simulink model "PV_ANN1"  (R2024b)
settings: Solver=ode23tb  StartTime=0.0  StopTime=3  MaxStep=1e-4  RelTol=1e-3
values from neighbouring files (symbols this model uses):
  TestID = testIDs(k)    [CloudMPPT_FullAnalytics.m]    (also in TestID.m = 0)
undefined symbols (not defined in the file or in its folder): MCS_ML_Selector_fun, sigbuilder_block
libraries: spsSeriesRLCBranchLib x3, spsDiodeLib x2, spsVoltageMeasurementLib x2, spsCurrentMeasurementLib x1, spsControlledCurrentSourceLib x1, spsIGBTLib x1, sps_lib x1, spsPWMGeneratorDCDCLib x1
(part 1 of 2)
settings Model: SimulationMode=accelerator  Creator=Ankita Arora  LastModifiedBy=qazvin
settings SolverCC: ZeroCrossAlgorithm=Adaptive  AlgebraicLoopSolver=TrustRegion
settings DataIOCC: SaveState=on  SignalLogging=off  ReturnWorkspaceOutputs=off
settings OptimizationCC: LifeSpan=inf
settings DebuggingCC: UnconnectedInputMsg=warning  UnconnectedOutputMsg=warning  UnconnectedLineMsg=warning  SFExecutionAtInitializationDiag=none  ArithmeticOperatorsInVariantConditions=warning
settings ModelReferenceCC: EnableRefExpFcnMdlSchedulingChecks=on
settings SFSimCC: SimUseLocalCustomCode=off  CustomCodeUndefinedFunction=UseInterfaceOnly
settings RTWCC: RTWUseLocalCustomCode=off  GPUComputeCapability=3.5
settings CodeAppCC: StateflowObjectComments=on
settings SimscapeCC: SimscapeNormalizeSystem=off

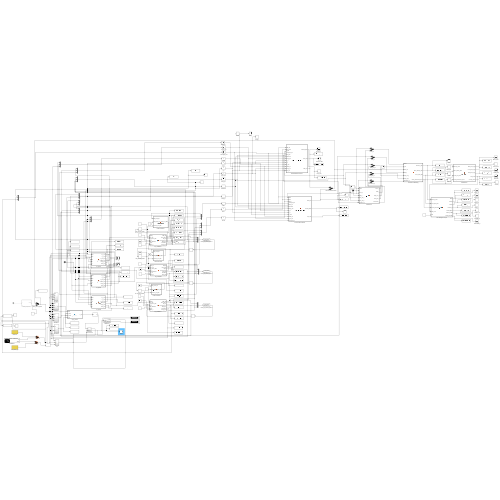
[thumbnail: Simulink's stored preview of the top-level diagram]
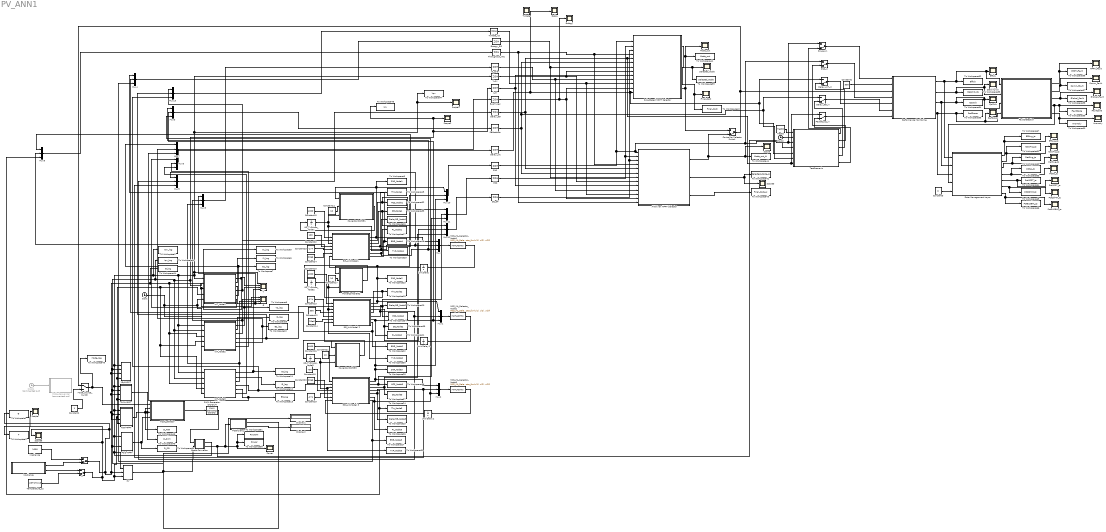
== system PV_ANN1 ==
  "      " : ManualSwitch  CurrentSetting=0
  "      1" : ManualSwitch  CurrentSetting=0
  " PacketLoss_in" : ManualSwitch  CurrentSetting=0
  " StabilityIdx   " : Scope
  5G_LinkModel 2 : MATLAB Function  TreatAsAtomicUnit=on
  "5G_LinkModel 3 " : MATLAB Function  TreatAsAtomicUnit=on
  "5G_LinkModel1 " : MATLAB Function  TreatAsAtomicUnit=on
  AI-Driven MPPT Selector : MATLAB Function  TreatAsAtomicUnit=on  SystemSampleTime=1e-4
  ANN-MPPT : Subsystem
  Anomaly : Scope
  Boost Convertor : Subsystem
  Clock : Clock
  Clock1 : Clock  Commented=on
  Clock2 : Clock
  Comm_Fault : Scope
  Constant1 : Constant
  Constant10 : Constant  Value=4000
  Constant11 : Constant  Value=10
  Constant12 : Constant  Value=300
  Constant13 : Constant  Value=-174
  Constant14 : Constant  Value=20e6
  Constant15 : Constant  Value=4000
  Constant16 : Constant  Value=4000
  Constant17 : Constant  Value=10
  Constant18 : Constant  Value=700
  Constant19 : Constant  Value=-174
  Constant2 : Constant  Value=500
  Constant20 : Constant  Value=20e6
  Constant21 : Constant  Value=10
  Constant22 : Constant  Value=100
  Constant23 : Constant  Value=-174
  Constant24 : Constant  Value=20e6
  Constant3 : Constant  Value=0
  Controller Selector Switch : ManualSwitch  CurrentSetting=0
  Data Management Layer : MATLAB Function  TreatAsAtomicUnit=on
  Delay : Scope
  Delay_5G : ZeroOrderHold  SampleTime=0.1
  Delay_5G_in : ManualSwitch  CurrentSetting=0
  Delay_IoT_in : ManualSwitch  CurrentSetting=0
  Delay_iot : ZeroOrderHold  SampleTime=0.1
  Display1 : Display
  Display2 : Display
  E_IoT_Vec : ZeroOrderHold  SampleTime=0.1
  EffAvg_ts : Scope
  EffIdx : Scope
  Energy : Scope
  Energy_5G : ZeroOrderHold  SampleTime=0.1
  FaultCode : Scope
  FaultDetection : MATLAB Function  TreatAsAtomicUnit=on
  Final_Cost : Scope
  G : Scope  NumInputPorts=4
  G_solar : ZeroOrderHold  SampleTime=0.1
  Global_Fault : Scope
  I_pv : ZeroOrderHold  SampleTime=0.1
  IoT_Node1 : MATLAB Function  TreatAsAtomicUnit=on  SystemSampleTime=0.01
  IoT_Node2 : MATLAB Function  TreatAsAtomicUnit=on  SystemSampleTime=0.02
  IoT_Node3 : MATLAB Function  TreatAsAtomicUnit=on  SystemSampleTime=0.05
  Irradiance : Constant  Value=1000
  "Irradiance " : Subsystem  Tag=STV Subsys  LoadFcn=sigbuilder_block('load');  StartFcn=sigbuilder_block('start');  StopFcn=sigbuilder_block('stop');  ClipboardFcn=sigbuilder_block('clipboard');  mask(Sigbuilder block){tuvar=[0:10]}
      mask help: Sigbuilder GUI
      mask init:
      | if ~strcmp(get_param(bdroot(gcbh),'SimulationStatus'),'stopped') tuvar = sigbuilder_block('maskInit'); end
      settings: CopyFcn=sigbuilder_block('copy');  DeleteFcn=sigbuilder_block('delete');  ModelCloseFcn=sigbuilder_block('modelClose');  PreSaveFcn=sigbuilder_block('preSave');  PauseFcn=sigbuilder_block('pause')  ContinueFcn=sigbuilder_block('continue')  NameChangeFcn=sigbuilder_block('namechange');  OpenFcn=sigbuilder_block('open',[5.4 30 1141.2 507.6 ]);  CloseFcn=sigbuilder_block('close');
      mask Display: plot(0, 0, 100, 100,[2, 2, 32, 32, 2], [68, 8, 8, 68, 68],[32, 2], [38, 38], [32, 19, 2],[53, 60, 44], [32, 17, 17, 2],[16, 16, 31, 31]);txt = getActiveGroup(gcbh);text(2, 100, txt,'verticalAlignment', 'top');
  MCS : ZeroOrderHold  SampleTime=0.1
  MCS_ML_Selector_Node1 : MATLABFcn  MATLABFcn=MCS_ML_Selector_fun(u(1), u(2), u(3))
  MCS_ML_Selector_Node2 : MATLABFcn  MATLABFcn=MCS_ML_Selector_fun(u(1), u(2), u(3))
  MCS_ML_Selector_Node3 : MATLABFcn  MATLABFcn=MCS_ML_Selector_fun(u(1), u(2), u(3))
  MPPT_Fault : Scope
  Mode_Sequencer : MATLAB Function  Commented=on  TreatAsAtomicUnit=on
  Mode_Source_Switch : ManualSwitch
  Mode_out : Scope
  Mux{,1..13} (14 alike) : Mux  Inputs=3
  P&Eficiency : Subsystem
  P&O-MPPT : Subsystem
  PV : Subsystem
  PWM Generator (DC-DC)4 : spsPWMGeneratorDCDCLib/PWM Generator (DC-DC)  Fsw=5000  Ts=0
  PacketLost : ZeroOrderHold  SampleTime=0.1
  PctCOMM_ts : Scope
  PctGLOBAL_ts : Scope
  PctMPPT_ts : Scope
  PctNo_ts : Scope
  PerfAvg_ts : Scope
  PerfScore : Scope
  Performance Monitoring : MATLAB Function  TreatAsAtomicUnit=on  SystemSampleTime=1e-4
  Power : Scope
  PowerControl5G1 : MATLAB Function  TreatAsAtomicUnit=on
  PowerControl5G2 : MATLAB Function  TreatAsAtomicUnit=on
  PowerControl5G3 : MATLAB Function  TreatAsAtomicUnit=on
  Power_in : ManualSwitch  CurrentSetting=0
  QoSAvg_ts : Scope
  QoSIdx : Scope
  Rule-Based MPPT Selector : MATLAB Function  TreatAsAtomicUnit=on  SystemSampleTime=1e-4
  SE_eff : ZeroOrderHold  SampleTime=0.1
  SNR : ZeroOrderHold  SampleTime=0.1
  SNR_in : ManualSwitch  CurrentSetting=0
  SVM-MPPT : Subsystem
  Scope{,1..3,6..7} (6 alike) : Scope
  Selected_Node : Scope
  Temperature_op : Constant  Value=25+273.15
  TestID : Constant  Value=TestID
  TestScenario : MATLAB Function  TreatAsAtomicUnit=on  SystemSampleTime=1e-4
  Throughput_Vec : ZeroOrderHold  SampleTime=0.1
  To Workspace : ToWorkspace  VariableName=G  SaveFormat=Timeseries  SampleTime=-1
  To Workspace1 : ToWorkspace  VariableName=T  SaveFormat=Timeseries  SampleTime=-1
  To Workspace10 : ToWorkspace  VariableName=E2_log  SampleTime=-1
  To Workspace11 : ToWorkspace  VariableName=V3_log  SampleTime=-1
  To Workspace12 : ToWorkspace  VariableName=I3_log  SampleTime=-1
  To Workspace13 : ToWorkspace  VariableName=E3_log  SampleTime=-1
  To Workspace14 : ToWorkspace  VariableName=G_log  SampleTime=-1
  To Workspace15 : ToWorkspace  VariableName=Thr_Node1  SampleTime=-1
  To Workspace16 : ToWorkspace  VariableName=Delay5G_Node1  SampleTime=-1
  To Workspace17 : ToWorkspace  VariableName=PL_Node1  SampleTime=-1
  To Workspace18 : ToWorkspace  VariableName=E5G_Node1  SampleTime=-1
  To Workspace19 : ToWorkspace  VariableName=Thr_Node2  SampleTime=-1
  To Workspace2 : ToWorkspace  VariableName=Vpv_log  SampleTime=-1
  To Workspace20 : ToWorkspace  VariableName=Delay5G_Node2  SampleTime=-1
  To Workspace21 : ToWorkspace  VariableName=PL_Node2  SampleTime=-1
  To Workspace22 : ToWorkspace  VariableName=E5G_Node2  SampleTime=-1
  To Workspace23 : ToWorkspace  VariableName=SNR_Node2  SampleTime=-1
  To Workspace24 : ToWorkspace  VariableName=Thr_Node3  SampleTime=-1
  To Workspace25 : ToWorkspace  VariableName=Delay5G_Node3  SampleTime=-1
  To Workspace26 : ToWorkspace  VariableName=PL_Node3  SampleTime=-1
  To Workspace27 : ToWorkspace  VariableName=E5G_Node3  SampleTime=-1
  To Workspace28 : ToWorkspace  VariableName=SNR_Node3  SampleTime=-1
  To Workspace29 : ToWorkspace  VariableName=TxP_Node1  SampleTime=-1
  To Workspace3 : ToWorkspace  VariableName=SNR_Node1  SampleTime=-1
  To Workspace30 : ToWorkspace  VariableName=TxP_Node2  SampleTime=-1
  To Workspace31 : ToWorkspace  VariableName=TxP_Node3  SampleTime=-1
  To Workspace32 : ToWorkspace  VariableName=MCS_Node1  SampleTime=-1
  To Workspace33 : ToWorkspace  VariableName=SE_Node1  SampleTime=-1
  To Workspace34 : ToWorkspace  VariableName=MCS_Node2  SampleTime=-1
  To Workspace35 : ToWorkspace  VariableName=SE_Node2  SampleTime=-1
  To Workspace36 : ToWorkspace  VariableName=MCS_Node3  SampleTime=-1
  To Workspace37 : ToWorkspace  VariableName=SE_Node3  SampleTime=-1
  To Workspace38 : ToWorkspace  VariableName=Power  SampleTime=5e-5
  To Workspace39 : ToWorkspace  VariableName=Selected_Node  SampleTime=-1
  To Workspace4 : ToWorkspace  VariableName=Ipv_log  SampleTime=-1
  To Workspace40 : ToWorkspace  VariableName=Final_Cost  SampleTime=-1
  To Workspace41 : ToWorkspace  VariableName=Mode_out  SampleTime=-1
  To Workspace42 : ToWorkspace  VariableName=Selected_Node_AI  SampleTime=-1
  To Workspace43 : ToWorkspace  VariableName=Final_Cost_AI  SampleTime=-1
  To Workspace44 : ToWorkspace  VariableName=Mode_out_AI  SampleTime=-1
  To Workspace45 : ToWorkspace  VariableName=Mode_log  SampleTime=-1
  To Workspace46 : ToWorkspace  VariableName=D_ANN  SampleTime=-1
  To Workspace47 : ToWorkspace  VariableName=Vpv  SaveFormat=Structure With Time  SampleTime=-1
  To Workspace48 : ToWorkspace  VariableName=Ipv  SaveFormat=Structure With Time  SampleTime=-1
  To Workspace49 : ToWorkspace  VariableName=D_SVM  SampleTime=-1
  To Workspace5 : ToWorkspace  VariableName=V1_log  SampleTime=-1
  To Workspace50 : ToWorkspace  VariableName=D_PO  SampleTime=-1
  To Workspace51 : ToWorkspace  VariableName=PowerAI  SampleTime=5e-5
  To Workspace52 : ToWorkspace  VariableName=EffIdx  SaveFormat=Timeseries  SampleTime=-1
  To Workspace53 : ToWorkspace  VariableName=StabilityIdx  SaveFormat=Timeseries  SampleTime=-1
  To Workspace54 : ToWorkspace  VariableName=QoSIdx  SaveFormat=Timeseries  SampleTime=-1
  To Workspace55 : ToWorkspace  VariableName=PerfScore  SaveFormat=Timeseries  SampleTime=-1
  To Workspace56 : ToWorkspace  VariableName=MPPT_Fault  SaveFormat=Timeseries  SampleTime=-1
  To Workspace57 : ToWorkspace  VariableName=Comm_Fault  SaveFormat=Timeseries  SampleTime=-1
  To Workspace58 : ToWorkspace  VariableName=Global_Fault  SaveFormat=Timeseries  SampleTime=-1
  To Workspace59 : ToWorkspace  VariableName=FaultCode  SaveFormat=Timeseries  SampleTime=-1
  To Workspace6 : ToWorkspace  VariableName=I1_log  SampleTime=-1
  To Workspace60 : ToWorkspace  VariableName=Anomaly  SaveFormat=Timeseries  SampleTime=-1
  To Workspace61 : ToWorkspace  VariableName=QoSAvg_ts  SaveFormat=Timeseries  SampleTime=-1
  To Workspace62 : ToWorkspace  VariableName=PerfAvg_ts  SaveFormat=Timeseries  SampleTime=-1
  To Workspace63 : ToWorkspace  VariableName=PctNo_ts  SaveFormat=Timeseries  SampleTime=-1
  To Workspace64 : ToWorkspace  VariableName=PctMPPT_ts  SaveFormat=Timeseries  SampleTime=-1
  To Workspace65 : ToWorkspace  VariableName=PctCOMM_ts  SaveFormat=Timeseries  SampleTime=-1
  To Workspace66 : ToWorkspace  VariableName=PctGLOBAL_ts  SaveFormat=Timeseries  SampleTime=-1
  To Workspace67 : ToWorkspace  VariableName=EffAvg_ts  SaveFormat=Timeseries  SampleTime=-1
  To Workspace7 : ToWorkspace  VariableName=E1_log  SampleTime=-1
  To Workspace8 : ToWorkspace  VariableName=V2_log  SampleTime=-1
  To Workspace9 : ToWorkspace  VariableName=I2_log  SampleTime=-1
  TxRate : Scope
  TxRate_iot : ZeroOrderHold  SampleTime=0.1
  UD_TxPower_Node1 : UnitDelay  SampleTime=-1  HasFrameUpgradeWarning=on
  UD_TxPower_Node2 : UnitDelay  SampleTime=-1  HasFrameUpgradeWarning=on
  UD_TxPower_Node3 : UnitDelay  SampleTime=-1  HasFrameUpgradeWarning=on
  Unit Delay : UnitDelay  SampleTime=-1  HasFrameUpgradeWarning=on
  Unit Delay1 : UnitDelay  SampleTime=-1  HasFrameUpgradeWarning=on
  Unit Delay2 : UnitDelay  SampleTime=-1  HasFrameUpgradeWarning=on
  V : Scope  NumInputPorts=4
  V5p-MPPT : Subsystem
  V_pv : ZeroOrderHold  SampleTime=0.1
  mppt_selector : MATLAB Function  TreatAsAtomicUnit=on
  wires:
  Temperature_op/1 -> "      1"/2
  Irradiance/1 -> "      "/1
  "      "/1 -> Scope6/1, To Workspace/1, PV/2(G), IoT_Node3/3(G), IoT_Node2/3(G), G/1, IoT_Node1/3(G), To Workspace14/1, V5p-MPPT/3(G), SVM-MPPT/3(G), ANN-MPPT/3(G)  "G"
  "      1"/1 -> To Workspace1/1, Scope7/1, PV/3(T), ANN-MPPT/4(T), IoT_Node3/4(T), IoT_Node2/4(T), IoT_Node1/4(T), V5p-MPPT/4(T), SVM-MPPT/4(T)  "T"
  PV/1(I) -> IoT_Node3/2(Ipv), IoT_Node2/2(Ipv), IoT_Node1/2(Ipv), To Workspace48/1, Scope2/1, I_pv/1, To Workspace4/1, V5p-MPPT/2(Ipv), SVM-MPPT/2(Ipv), ANN-MPPT/2(Ipv), P&O-MPPT/2(Ipv), Boost Convertor/2(s)
  P&O-MPPT/1(D) -> To Workspace50/1, mppt_selector/4(D_PO)
  mppt_selector/1(D_ref) -> PWM Generator (DC-DC)4/1
  Boost Convertor/1(v) -> PV/1(V), IoT_Node3/1(Vpv), IoT_Node2/1(Vpv), V/1, To Workspace47/1, Scope1/1, V_pv/1, IoT_Node1/1(Vpv), To Workspace2/1, V5p-MPPT/1(Vpv), SVM-MPPT/1(Vpv), ANN-MPPT/1(Vpv), P&O-MPPT/1(Vpv)
  PWM Generator (DC-DC)4/1 -> Boost Convertor/1(g)
  P&Eficiency/1(Pmax) -> Display1/1
  P&Eficiency/2(max_efficiency) -> Display2/1
  IoT_Node1/1(V_pv_iot1) -> V/2, To Workspace5/1
  IoT_Node2/1(V_pv_iot2) -> To Workspace8/1, V/3
  IoT_Node3/1(V_pv_iot3) -> To Workspace11/1, V/4
  IoT_Node1/3(G_solar_iot1) -> Mux9/1, G/4
  IoT_Node3/3(G_solar_iot3) -> Mux9/3, G/3
  IoT_Node2/3(G_solar_iot2) -> Mux9/2, G/2
  IoT_Node3/2(I_pv_iot3) -> To Workspace12/1
  IoT_Node3/5(Energy_iot3) -> To Workspace13/1, Mux7/3
  IoT_Node2/5(Energy_iot2) -> Mux7/2, To Workspace10/1
  IoT_Node2/2(I_pv_iot2) -> To Workspace9/1
  IoT_Node1/5(Energy_iot1) -> Mux7/1, To Workspace7/1
  IoT_Node1/2(I_pv_iot1) -> To Workspace6/1
  Clock/1 -> IoT_Node1/5(t), IoT_Node2/5(t), IoT_Node3/5(t)
  IoT_Node1/4(TxRate_iot1) -> Mux13/1, "5G_LinkModel1 "/2(IoT_rate)
  Constant18/1 -> "5G_LinkModel 3 "/4(d_m)
  Constant19/1 -> "5G_LinkModel 3 "/5(N0_dBmPerHz)
  Constant20/1 -> "5G_LinkModel 3 "/6(B_Hz)
  Constant15/1 -> "5G_LinkModel1 "/1(Data_in)
  Constant22/1 -> "5G_LinkModel1 "/4(d_m)
  Constant23/1 -> "5G_LinkModel1 "/5(N0_dBmPerHz)
  Constant24/1 -> "5G_LinkModel1 "/6(B_Hz)
  IoT_Node2/4(TxRate_iot2) -> Mux13/2, 5G_LinkModel 2/2(IoT_rate)
  Constant10/1 -> 5G_LinkModel 2/1(Data_in)
  Constant12/1 -> 5G_LinkModel 2/4(d_m)
  Constant13/1 -> 5G_LinkModel 2/5(N0_dBmPerHz)
  Constant14/1 -> 5G_LinkModel 2/6(B_Hz)
  IoT_Node3/4(TxRate_iot3) -> Mux13/3, "5G_LinkModel 3 "/2(IoT_rate)
  Constant16/1 -> "5G_LinkModel 3 "/1(Data_in)
  "5G_LinkModel1 "/1(SNR_dB) -> Mux/1, PowerControl5G1/1(SNR_meas_dB), To Workspace3/1, Mux10/1
  "5G_LinkModel1 "/5(Delay_5G) -> Mux5/1, Mux/2, To Workspace16/1
  "5G_LinkModel1 "/6(PacketLost) -> Mux/3, Mux3/1, To Workspace17/1
  "5G_LinkModel1 "/7(Energy_5G) -> Mux4/1, To Workspace18/1
  5G_LinkModel 2/1(SNR_dB) -> PowerControl5G2/1(SNR_meas_dB), Mux10/2, To Workspace23/1, Mux1/1
  5G_LinkModel 2/5(Delay_5G) -> Mux5/2, Mux1/2, To Workspace20/1
  5G_LinkModel 2/6(PacketLost) -> Mux3/2, Mux1/3, To Workspace21/1
  5G_LinkModel 2/7(Energy_5G) -> Mux4/2, To Workspace22/1
  "5G_LinkModel 3 "/7(Energy_5G) -> Mux4/3, To Workspace27/1
  "5G_LinkModel 3 "/6(PacketLost) -> Mux3/3, Mux2/3, To Workspace26/1
  "5G_LinkModel 3 "/5(Delay_5G) -> To Workspace25/1, Mux5/3, Mux2/2
  "5G_LinkModel 3 "/1(SNR_dB) -> Mux10/3, PowerControl5G3/1(SNR_meas_dB), To Workspace28/1, Mux2/1
  UD_TxPower_Node3/1 -> To Workspace31/1, "5G_LinkModel 3 "/3(Tx_Power_dBm), PowerControl5G3/3(TxPower_prev_dBm)
  UD_TxPower_Node1/1 -> To Workspace29/1, "5G_LinkModel1 "/3(Tx_Power_dBm), PowerControl5G1/3(TxPower_prev_dBm)
  UD_TxPower_Node2/1 -> To Workspace30/1, 5G_LinkModel 2/3(Tx_Power_dBm), PowerControl5G2/3(TxPower_prev_dBm)
  PowerControl5G3/1(TxPower_out_dBm) -> UD_TxPower_Node3/1
  PowerControl5G1/1(TxPower_out_dBm) -> UD_TxPower_Node1/1
  PowerControl5G2/1(TxPower_out_dBm) -> UD_TxPower_Node2/1
  Constant11/1 -> PowerControl5G1/2(SNR_target_dB)
  Constant17/1 -> PowerControl5G2/2(SNR_target_dB)
  Constant21/1 -> PowerControl5G3/2(SNR_target_dB)
  "5G_LinkModel1 "/4(Throughput_bps) -> Mux8/1, To Workspace15/1
  5G_LinkModel 2/4(Throughput_bps) -> Mux8/2, To Workspace19/1
  "5G_LinkModel 3 "/4(Throughput_bps) -> Mux8/3, To Workspace24/1
  "5G_LinkModel 3 "/2(MCS_index) -> Mux11/3, To Workspace36/1
  "5G_LinkModel 3 "/3(SE_eff) -> To Workspace37/1, Mux12/3
  5G_LinkModel 2/2(MCS_index) -> To Workspace34/1, Mux11/2
  "5G_LinkModel1 "/3(SE_eff) -> Mux12/1, To Workspace33/1
  "5G_LinkModel1 "/2(MCS_index) -> Mux11/1, To Workspace32/1
  Mux/1 -> MCS_ML_Selector_Node1/1
  Mux1/1 -> MCS_ML_Selector_Node2/1
  Mux2/1 -> MCS_ML_Selector_Node3/1
  MCS_ML_Selector_Node3/1 -> Unit Delay2/1
  MCS_ML_Selector_Node2/1 -> Unit Delay1/1
  MCS_ML_Selector_Node1/1 -> Unit Delay/1
  Unit Delay/1 -> "5G_LinkModel1 "/7(MCS_in)
  Unit Delay1/1 -> 5G_LinkModel 2/7(MCS_in)
  Unit Delay2/1 -> "5G_LinkModel 3 "/7(MCS_in)
  IoT_Node1/6(Delay_iot1) -> Mux6/1
  IoT_Node2/6(Delay_iot2) -> Mux6/2
  IoT_Node3/6(Delay_iot3) -> Mux6/3
  Mux7/1 -> E_IoT_Vec/1
  Mux4/1 -> Energy_5G/1
  Mux5/1 -> Delay_5G/1
  Mux3/1 -> PacketLost/1
  Mux8/1 -> Throughput_Vec/1
  ANN-MPPT/1(D) -> To Workspace46/1, mppt_selector/2(D_ANN)
  SVM-MPPT/1(D) -> To Workspace49/1, mppt_selector/3(D_SVM)
  I_pv/1 -> AI-Driven MPPT Selector/9(I_pv), Rule-Based MPPT Selector/9(I_pv)
  Throughput_Vec/1 -> AI-Driven MPPT Selector/13(Throughput_iot), AI-Driven MPPT Selector/4(Throughput_Vec), Rule-Based MPPT Selector/4(Throughput_bps)
  E_IoT_Vec/1 -> AI-Driven MPPT Selector/12(E_IoT_Vec), Rule-Based MPPT Selector/12(Energy_iot), Energy/1
  Energy_5G/1 -> AI-Driven MPPT Selector/7(Energy_5G), Rule-Based MPPT Selector/7(Energy_5G)
  V_pv/1 -> AI-Driven MPPT Selector/8(V_pv), Rule-Based MPPT Selector/8(V_pv)
  Mux9/1 -> G_solar/1
  G_solar/1 -> AI-Driven MPPT Selector/10(G_solar), Rule-Based MPPT Selector/10(G_solar)
  Delay_5G/1 -> AI-Driven MPPT Selector/5(Delay_5G), " PacketLoss_in"/1, TestScenario/7(PacketLoss_in), Rule-Based MPPT Selector/5(Delay_5G)
  Mux6/1 -> Delay_iot/1
  Delay_iot/1 -> Delay/1, TestScenario/5(Delay_IoT_in), Delay_IoT_in/1, Rule-Based MPPT Selector/13(Delay_iot)
  Mux10/1 -> SNR/1
  SNR/1 -> Rule-Based MPPT Selector/1(SNR_dB), SNR_in/1, TestScenario/4(SNR_in), AI-Driven MPPT Selector/1(SNR)
  Mux11/1 -> MCS/1
  MCS/1 -> Rule-Based MPPT Selector/2(MCS_index), AI-Driven MPPT Selector/2(MCS)
  5G_LinkModel 2/3(SE_eff) -> Mux12/2, To Workspace35/1
  Mux12/1 -> SE_eff/1
  SE_eff/1 -> Rule-Based MPPT Selector/3(SE_eff), AI-Driven MPPT Selector/3(SE_eff)
  Rule-Based MPPT Selector/3(Mode_out) -> Mode_out/1, To Workspace41/1, Controller Selector Switch/1
  Rule-Based MPPT Selector/2(Final_Cost) -> To Workspace40/1, Final_Cost/1
  "Irradiance "/1(G) -> "      "/2
  "Irradiance "/2(Temp) -> "      1"/1
  Mux13/1 -> TxRate_iot/1
  Rule-Based MPPT Selector/1(Selected_Node) -> To Workspace39/1, Selected_Node/1
  TxRate_iot/1 -> AI-Driven MPPT Selector/11(TxRate_iot), Rule-Based MPPT Selector/11(TxRate_iot)
  AI-Driven MPPT Selector/1(Mode_out) -> Controller Selector Switch/2, Scope/1, To Workspace44/1
  AI-Driven MPPT Selector/3(Final_Cost) -> To Workspace43/1
  AI-Driven MPPT Selector/2(Selected_Node) -> To Workspace42/1, Scope3/1
  Clock1/1 -> Mode_Sequencer/1(t)
  Controller Selector Switch/1 -> Performance Monitoring/3(Mode_out), Mode_Source_Switch/1
  Mode_Source_Switch/1 -> To Workspace45/1, mppt_selector/1(Mode)
  Constant1/1 -> Mode_Source_Switch/2
  Constant2/1 -> Performance Monitoring/2(P_ref)
  Performance Monitoring/1(Efficiency_Index) -> Data Management Layer/1(Efficiency_Index), FaultDetection/1(Efficiency_Index), EffIdx/1, To Workspace52/1
  Performance Monitoring/2(MPPT_Stability_Index) -> " StabilityIdx   "/1, FaultDetection/2(MPPT_Stability_Index), To Workspace53/1
  Performance Monitoring/3(Comm_QoS_Index) -> Data Management Layer/2(Comm_QoS_Index), FaultDetection/3(Comm_QoS_Index), QoSIdx/1, To Workspace54/1
  Performance Monitoring/4(Overall_Performance_Score) -> Data Management Layer/3(Overall_Performance_Score), PerfScore/1, FaultDetection/4(Overall_Performance_Score), To Workspace55/1
  FaultDetection/1(MPPT_Fault_Flag) -> To Workspace56/1, MPPT_Fault/1
  FaultDetection/2(Comm_Fault_Flag) -> Comm_Fault/1, To Workspace57/1
  FaultDetection/3(Global_Fault_Flag) -> Global_Fault/1, To Workspace58/1
  FaultDetection/4(Fault_Code) -> Data Management Layer/4(Fault_Code), FaultCode/1, To Workspace59/1
  FaultDetection/5(Anomaly_Score) -> Anomaly/1, To Workspace60/1
  PacketLost/1 -> Rule-Based MPPT Selector/6(PacketLost), TestScenario/6(Delay_5G_in), Delay_5G_in/1, AI-Driven MPPT Selector/6(PacketLost)
  TestID/1 -> TestScenario/1(TestID)
  Clock2/1 -> TestScenario/2(t)
  Power_in/1 -> Performance Monitoring/1(Power)
  Boost Convertor/2(PVPower) -> Power_in/1, TestScenario/3(Power_in), To Workspace51/1, To Workspace38/1, Power/1, P&Eficiency/1(P_out)
  TestScenario/1(Power_t) -> Power_in/2
  SNR_in/1 -> Performance Monitoring/4(SNR_in)
  TestScenario/2(SNR_t) -> SNR_in/2
  Delay_IoT_in/1 -> Performance Monitoring/5(Delay_IoT_in)
  " PacketLoss_in"/1 -> Performance Monitoring/7(PacketLoss_in)
  Delay_5G_in/1 -> Performance Monitoring/6(Delay_5G_in)
  TestScenario/5(PacketLoss_t) -> " PacketLoss_in"/2
  TestScenario/4(Delay_5G_t) -> Delay_5G_in/2
  TestScenario/3(Delay_IoT_t) -> Delay_IoT_in/2
  Constant3/1 -> Data Management Layer/5(reset)
  Data Management Layer/1(EffAvg) -> To Workspace67/1, EffAvg_ts/1
  Data Management Layer/2(QoSAvg) -> To Workspace61/1, QoSAvg_ts/1
  Data Management Layer/3(PerfAvg) -> To Workspace62/1, PerfAvg_ts/1
  Data Management Layer/4(FaultPct_No) -> To Workspace63/1, PctNo_ts/1
  Data Management Layer/5(FaultPct_MPPT) -> PctMPPT_ts/1, To Workspace64/1
  Data Management Layer/6(FaultPct_COMM) -> PctCOMM_ts/1, To Workspace65/1
  Data Management Layer/7(FaultPct_GLOBAL) -> PctGLOBAL_ts/1, To Workspace66/1

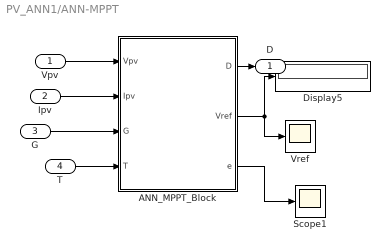
== system PV_ANN1/ANN-MPPT ==
  Vpv : Inport
  Ipv : Inport  Port=2
  G : Inport  Port=3
  T : Inport  Port=4
  ANN_MPPT_Block : MATLAB Function  TreatAsAtomicUnit=on  SystemSampleTime=1e-4
  Display5 : Display
  Scope1 : Scope
  Vref : Scope
  D : Outport
  wires:
  Ipv/1 -> ANN_MPPT_Block/2(Ipv)
  ANN_MPPT_Block/1(D) -> D/1
  T/1 -> ANN_MPPT_Block/4(T)
  ANN_MPPT_Block/2(Vref) -> Vref/1, Display5/1
  G/1 -> ANN_MPPT_Block/3(G)
  ANN_MPPT_Block/3(e) -> Scope1/1
  Vpv/1 -> ANN_MPPT_Block/1(Vpv)

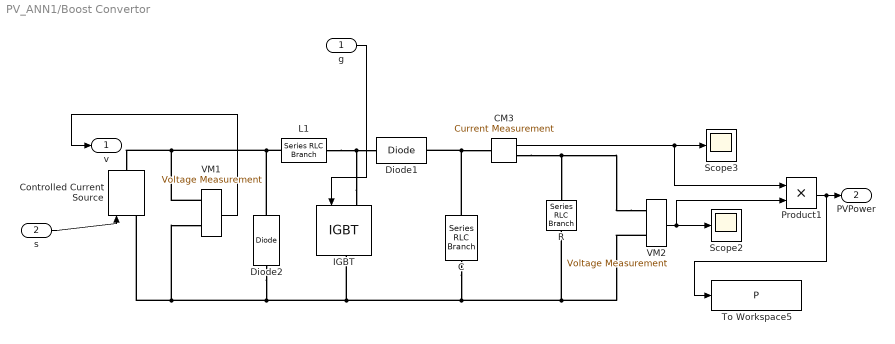
== system PV_ANN1/Boost Convertor ==
  g : Inport
  s : Inport  Port=2
  C : spsSeriesRLCBranchLib/Series RLC Branch  LConnTagsString=__new0  RConnTagsString=__new0  BranchType=C  Resistance=0.01  Inductance=1.0  SetiL0=off  InitialCurrent=0  Capacitance=3e-03  Setx0=off  InitialVoltage=200  Measurements=None
  CM3 : spsCurrentMeasurementLib/Current Measurement  Tag=PoWeRsYsTeMmEaSuReMeNt  PhasorSimulation=off  OutputType=Magnitude  PSBequivalent=0
      settings: AttributesFormatString=\n
  Controlled Current Source : spsControlledCurrentSourceLib/Controlled Current Source  Initialize=on  Source_Type=AC  Amplitude=0  Phase=0  Frequency=0  Measurements=None
  Diode1 : spsDiodeLib/Diode  Ron=0.001  Lon=0  Vf=0.8  IC=0  UseSnubber=off  Rs=500  Cs=250e-9  Measurements=off
      settings: AttributesFormatString=\n
  Diode2 : spsDiodeLib/Diode  Ron=0.001  Lon=0  Vf=0.8  IC=0  UseSnubber=off  Rs=500  Cs=250e-9  Measurements=off
      settings: AttributesFormatString=\n
  IGBT : spsIGBTLib/IGBT  Ron=0.001  Lon=0  Vf=1  Tf=1e-6  Tt=2e-6  IC=0  Rs=1e5  Cs=inf  Measurements=off
  L1 : spsSeriesRLCBranchLib/Series RLC Branch  LConnTagsString=__new0  RConnTagsString=__new0  BranchType=L  Resistance=1.0  Inductance=8.5e-03  SetiL0=off  InitialCurrent=0  Capacitance=1.0  Setx0=off  InitialVoltage=0  Measurements=None
  Product1 : Product  RndMeth=Zero
  R : spsSeriesRLCBranchLib/Series RLC Branch  LConnTagsString=__new0  RConnTagsString=__new0  BranchType=R  Resistance=40  Inductance=1.0  SetiL0=off  InitialCurrent=0  Capacitance=1.0  Setx0=off  InitialVoltage=0  Measurements=None
  Scope2 : Scope
  Scope3 : Scope
  To Workspace5 : ToWorkspace  VariableName=P  SaveFormat=Timeseries  SampleTime=-1
  VM1 : spsVoltageMeasurementLib/Voltage Measurement  Tag=PoWeRsYsTeMmEaSuReMeNt  PhasorSimulation=off  OutputType=Magnitude  PSBequivalent=0
  VM2 : spsVoltageMeasurementLib/Voltage Measurement  Tag=PoWeRsYsTeMmEaSuReMeNt  PhasorSimulation=off  OutputType=Magnitude  PSBequivalent=0
  v : Outport
  PVPower : Outport  Port=2
  wires:
  VM1/1 -> v/1
  CM3/1 -> Product1/1, Scope3/1
  Product1/1 -> To Workspace5/1, PVPower/1
  VM2/1 -> Product1/2, Scope2/1
  g/1 -> IGBT/1
  s/1 -> Controlled Current Source/1
  connections:
  Diode1/RConn1 -- C/LConn1 -- CM3/LConn1
  C/RConn1 -- VM2/LConn2 -- R/RConn1 -- IGBT/RConn1 -- Diode2/LConn1 -- Controlled Current Source/LConn1 -- VM1/LConn2
  VM1/LConn1 -- Diode2/RConn1 -- L1/LConn1 -- Controlled Current Source/RConn1
  IGBT/LConn1 -- L1/RConn1 -- Diode1/LConn1
  VM2/LConn1 -- CM3/RConn1 -- R/LConn1

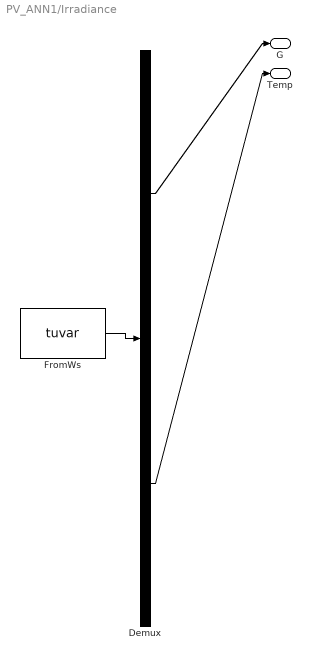
== system PV_ANN1/Irradiance  ==
  Demux : Demux  Tag=STV Demux  Outputs=2
      settings: DisplayOption=none
  FromWs : FromWorkspace  Tag=STV FromWs  VariableName=tuvar
      SigBuilderData=|
      | common.afterFinalStr = 'Extrapolate'
      | common.sampleTime = '0'
      | dataSet(1).timeRange = [0 2]
      | dataSet(1).name = 'Constant Irradiance'
      | dataSet(2).timeRange = [0 2]
      | dataSet(2).name = 'Step Irradiance'
      | dataSet(3).timeRange = [0 3]
      | dataSet(3).name = 'Ramp-up/down Irradiance'
      | sbobj.Groups(1).Name = 'Constant Irradiance'
      | sbobj.Groups(1).Signals(1).Name = 'G'
      | sbobj.Groups(1).Signals(1).XData = [0 2]
      | sbobj.Groups(1).Signals(1).YData = [1000 1000]
      | sbobj.Groups(1).Signals(2).Name = 'Temp'
      | sbobj.Groups(1).Signals(2).XData = [0 1 1 2]
      | sbobj.Groups(1).Signals(2).YData = [0 0 1 1]
      | sbobj.Groups(1).TimeRange = [0 2]
      | sbobj.Groups(2).Name = 'Step Irradiance'
      | sbobj.Groups(2).Signals(1).Name = 'G'
      | sbobj.Groups(2).Signals(1).XData = [0 0.252 0.252 2]
      | sbobj.Groups(2).Signals(1).YData = [600 600 1000 1000]
      | sbobj.Groups(2).Signals(2).Name = 'Temp'
      | sbobj.Groups(2).Signals(2).XData = [0 1 1 2]
      | sbobj.Groups(2).Signals(2).YData = [0 0 1 1]
      | sbobj.Groups(2).TimeRange = [0 2]
      | sbobj.Groups(3).Name = 'Ramp-up/down Irradiance'
      | sbobj.Groups(3).Signals(1).Name = 'G'
      | sbobj.Groups(3).Signals(1).XData = [0 0.75 0.75 1.5 1.5 2.25 2.25 3]
      | sbobj.Groups(3).Signals(1).YData = [1000 1000 800 800 600 600 1000 1000]
      | sbobj.Groups(3).Signals(2).Name = 'Temp'
      | sbobj.Groups(3).Signals(2).XData = [0 3]
      | sbobj.Groups(3).Signals(2).YData = [25 25]
      | sbobj.Groups(3).TimeRange = [0 3]
  G : Outport  Tag=STV Outport
  Temp : Outport  Tag=STV Outport  Port=2
  wires:
  Demux/1 -> G/1
  FromWs/1 -> Demux/1
  Demux/2 -> Temp/1

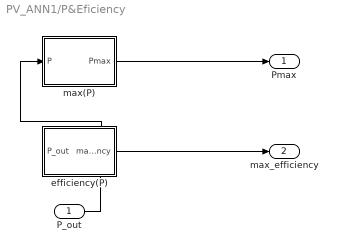
== system PV_ANN1/P&Eficiency ==
  P_out : Inport
  efficiency(P) : MATLAB Function  TreatAsAtomicUnit=on  SystemSampleTime=1e-4
  max(P) : MATLAB Function  TreatAsAtomicUnit=on  SystemSampleTime=1e-4
  Pmax : Outport
  max_efficiency : Outport  Port=2
  wires:
  P_out/1 -> max(P)/1(P), efficiency(P)/1(P_out)
  efficiency(P)/1(max_efficiency) -> max_efficiency/1
  max(P)/1(Pmax) -> Pmax/1

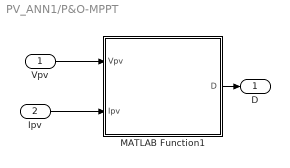
== system PV_ANN1/P&O-MPPT ==
  Vpv : Inport
  Ipv : Inport  Port=2
  MATLAB Function1 : MATLAB Function  TreatAsAtomicUnit=on  SystemSampleTime=1e-3
  D : Outport
  wires:
  Ipv/1 -> MATLAB Function1/2(Ipv)
  MATLAB Function1/1(D) -> D/1
  Vpv/1 -> MATLAB Function1/1(Vpv)

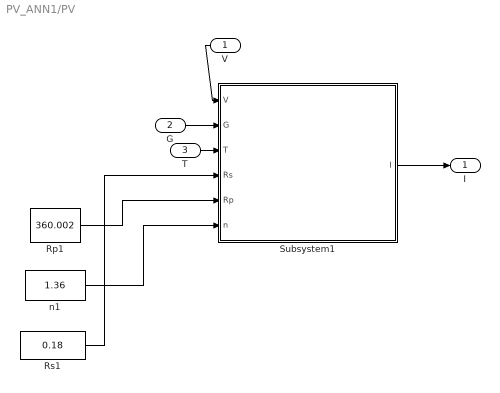
== system PV_ANN1/PV ==
  V : Inport
  G : Inport  Port=2
  T : Inport  Port=3
  Rp1 : Constant  Value=360.002
  Rs1 : Constant  Value=0.18
  Subsystem1 : Subsystem
  n1 : Constant  Value=1.36
  I : Outport
  wires:
  V/1 -> Subsystem1/1(V)
  Rp1/1 -> Subsystem1/5(Rp)
  Rs1/1 -> Subsystem1/4(Rs)
  Subsystem1/1(I) -> I/1
  G/1 -> Subsystem1/2(G)
  n1/1 -> Subsystem1/6(n)
  T/1 -> Subsystem1/3(T)

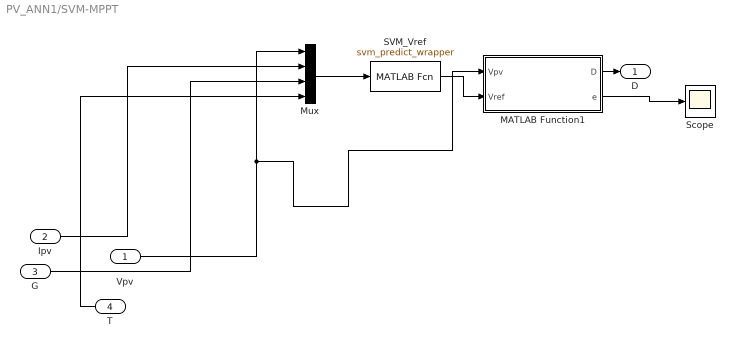
== system PV_ANN1/SVM-MPPT ==
  Vpv : Inport
  Ipv : Inport  Port=2
  G : Inport  Port=3
  T : Inport  Port=4
  MATLAB Function1 : MATLAB Function  TreatAsAtomicUnit=on  SystemSampleTime=1e-4
  Mux : Mux
  SVM_Vref : MATLABFcn  MATLABFcn=svm_predict_wrapper  OutputDimensions=1
  Scope : Scope
  D : Outport
  wires:
  SVM_Vref/1 -> MATLAB Function1/2(Vref)
  Mux/1 -> SVM_Vref/1
  G/1 -> Mux/3
  Vpv/1 -> Mux/1, MATLAB Function1/1(Vpv)
  MATLAB Function1/2(e) -> Scope/1
  T/1 -> Mux/4
  MATLAB Function1/1(D) -> D/1
  Ipv/1 -> Mux/2

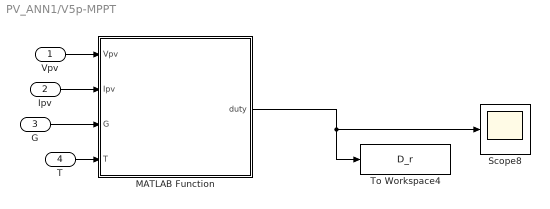
== system PV_ANN1/V5p-MPPT ==
  Vpv : Inport
  Ipv : Inport  Port=2
  G : Inport  Port=3
  T : Inport  Port=4
  MATLAB Function : MATLAB Function  TreatAsAtomicUnit=on  SystemSampleTime=1e-4
  Scope8 : Scope
  To Workspace4 : ToWorkspace  VariableName=D_r  SaveFormat=Timeseries  SampleTime=-1
  wires:
  Vpv/1 -> MATLAB Function/1(Vpv)
  MATLAB Function/1(duty) -> To Workspace4/1, Scope8/1
  T/1 -> MATLAB Function/4(T)
  G/1 -> MATLAB Function/3(G)
  Ipv/1 -> MATLAB Function/2(Ipv)

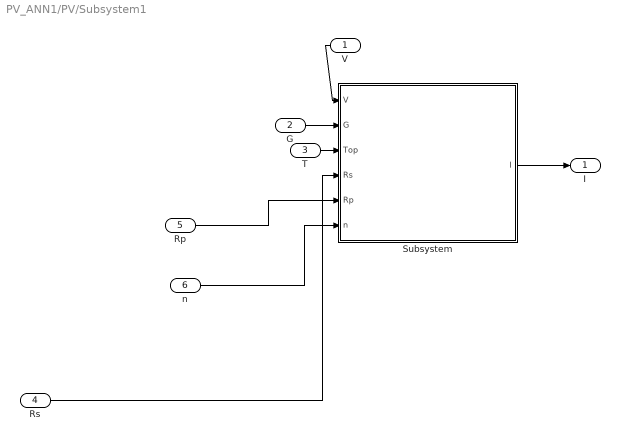
== system PV_ANN1/PV/Subsystem1 ==
  V : Inport
  G : Inport  Port=2
  T : Inport  Port=3
  Rs : Inport  Port=4
  Rp : Inport  Port=5
  n : Inport  Port=6
  Subsystem : Subsystem
  I : Outport
  wires:
  G/1 -> Subsystem/2(G)
  Rp/1 -> Subsystem/5(Rp)
  Subsystem/1(I) -> I/1
  n/1 -> Subsystem/6(n)
  V/1 -> Subsystem/1(V)
  Rs/1 -> Subsystem/4(Rs)
  T/1 -> Subsystem/3(Top)

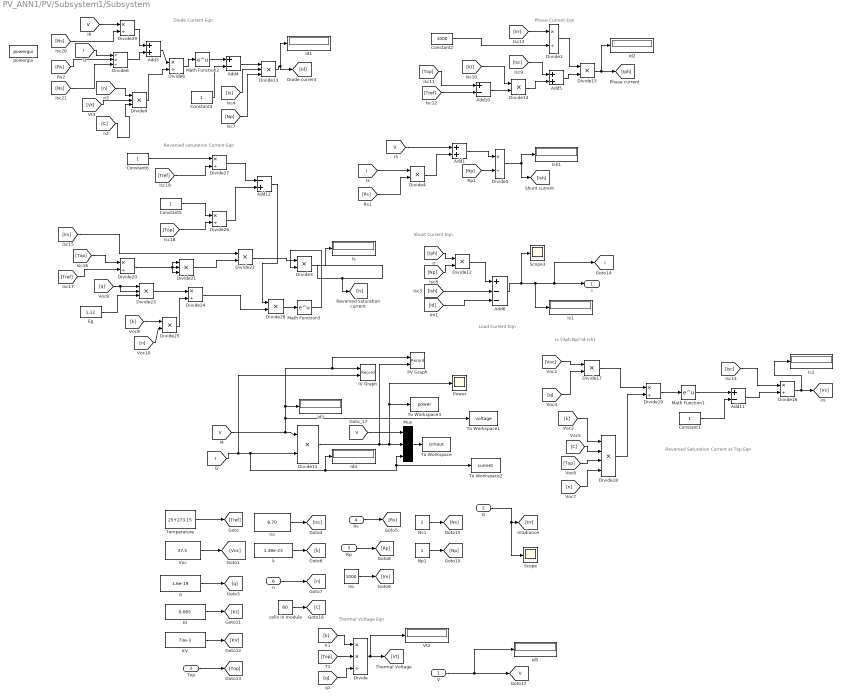
== system PV_ANN1/PV/Subsystem1/Subsystem ==
  note: Diode Current Eqn
  note: Shunt Current Eqn
  note: Phase Current Eqn
  note: Reversed saturation Current Eqn
  note: Load Current Eqn
  note: I={(Iph.Np)-Id-Ish}
  note: Reversed Saturation Current at Top Eqn
  note: Thermal Voltage Eqn
  V : Inport
  G : Inport  Port=2
  Top : Inport  Port=3
  Rs : Inport  Port=4
  Rp : Inport  Port=5
  n : Inport  Port=6
  Add1 : Sum
  Add10 : Sum  Inputs=+-
  Add11 : Sum  Inputs=+-
  Add12 : Sum  Inputs=-+
  Add3 : Sum
  Add4 : Sum  Inputs=+-
  Add5 : Sum
  Add6 : Sum  Inputs=+--
  Constant{1,3,5..6} (4 alike) : Constant
  Constant2 : Constant  Value=1000
  Divide : Product  Inputs=**/
  Divide{1,5..6,16,19..20,24,26..27,29} (10 alike) : Product  Inputs=*/
  Divide{3..4,11..12,14..15,17,22,25,28} (10 alike) : Product  Inputs=**
  Divide{9,13,21,23} (4 alike) : Product  Inputs=***
  Divide18 : Product  Inputs=****
  Divide8 : Product  Inputs=**/
  Eg : Constant  Value=1.12
  IV Graph : Record  FileSettingsInternal="{\"entries\":[{\"content\":{\"excelSettings\":{\"content\":{},\"type\":\"Streamout.ExcelSettings\"}},\"type\":\"Streamout.FileSettingStorage\",\"uuid\":\"\"}],\"packageUris\":[\"http:\\/\\/schema.mathworks.com\\/mf0\\/streamout_blocks\\/R2020a\"],\"version\":\"1.0\"}"  Layout=[1 1]  SignalsInternal="{\"entries\":[{\"content\":{\"signals\":[{\"content\":{\"blockPath\":[],\"dimensions\":[1],\"domain\":\"\",\"lineColor\":\"#139fff\",\"lineWidth\":2,\"port\":1,\"sid\":[\"\"],\"signalID\":1,\"signalName\":\"I4\"},\"type\":\"RecordBlkView.Signal\",\"uuid\":\"\"},{\"content\":{\"blockPath\":[],\"dimensions\":[1],\"domain\":\"\",\"lineColor\":\"#ff6929\",\"lineWidth\":2,\"port\":2,\"sid\":[\"\"],\"signalID\":2,\"signalName\":\"I2\"},\"type\":\"RecordBlkView.Signal\",\"uuid\":\"\"}]},\"type\":\"RecordBlkView.InputSignals\",\"uuid\":\"\"}],\"packageUris\":[\"http:\\/\\/schema.mathworks.com\\/mf0\\/streamout_blocks\\/R2020a\"],\"version\":\"1.0\"}"  VisualizationBindings="{\"xyplotplugin\":{\"info\":[{\"series\":[],\"subplotID\":1}]}}"  CompatibilityTag=XY  st=-1
  Id{1..5} (5 alike) : Display
  Iro : Constant  Value=1000
  Is : Display
  Is1 : Display
  Is2 : Display
  Isc : Constant  Value=8.70
  Ish1 : Display
  KI : Constant  Value=0.065
  KV : Constant  Value=73e-3
  Math Function1 : Math  SignedPower=on
  Math Function2 : Math  SignedPower=on
  Math Function3 : Math  SignedPower=on
  Mux : Mux  Inputs=3
  Np1 : Constant
  Ns1 : Constant  Value=2
  PV Graph : Record  FileSettingsInternal="{\"entries\":[{\"content\":{\"excelSettings\":{\"content\":{},\"type\":\"Streamout.ExcelSettings\"}},\"type\":\"Streamout.FileSettingStorage\",\"uuid\":\"\"}],\"packageUris\":[\"http:\\/\\/schema.mathworks.com\\/mf0\\/streamout_blocks\\/R2020a\"],\"version\":\"1.0\"}"  Layout=[1 1]  SignalsInternal="{\"entries\":[{\"content\":{\"signals\":[{\"content\":{\"blockPath\":[],\"dimensions\":[1],\"domain\":\"\",\"lineColor\":\"#b746ff\",\"lineWidth\":2,\"port\":1,\"sid\":[\"\"],\"signalID\":1,\"signalName\":\"I4\"},\"type\":\"RecordBlkView.Signal\",\"uuid\":\"\"},{\"content\":{\"blockPath\":[],\"dimensions\":[1],\"domain\":\"\",\"lineColor\":\"#64d413\",\"lineWidth\":2,\"port\":2,\"sid\":[\"\"],\"signalID\":2,\"signalName\":\"Divide11\"},\"type\":\"RecordBlkView.Signal\",\"uuid\":\"\"}]},\"type\":\"RecordBlkView.InputSignals\",\"uuid\":\"\"}],\"packageUris\":[\"http:\\/\\/schema.mathworks.com\\/mf0\\/streamout_blocks\\/R2020a\"],\"version\":\"1.0\"}"  VisualizationBindings="{\"xyplotplugin\":{\"info\":[{\"series\":[],\"subplotID\":1}]}}"  CompatibilityTag=XY  st=-1
  Power : Scope
  Scope : Scope
  Scope3 : Scope
  Temperature : Constant  Value=25+273.15
  To Workspace : ToWorkspace  VariableName=simout  SampleTime=-1
  To Workspace1 : ToWorkspace  VariableName=voltage  SampleTime=-1
  To Workspace2 : ToWorkspace  VariableName=current  SampleTime=-1
  To Workspace3 : ToWorkspace  VariableName=power  SampleTime=-1
  Voc : Constant  Value=37.5
  Vt2 : Display
      settings: Format=long_e
  cells in module : Constant  Value=60
  k : Constant  Value=1.38e-23
  powergui : sps_lib/powergui  SimulationMode=Continuous  SampleTime=50e-6  frequency=60  Iterations=50  frequencyindice=0  Pbase=100e6  ErrMax=1e-4  UnitsV=kV  UnitsW=MW  buscounter=0  FunctionMessages=off  echomessages=off  EnableUseOfTLC=off  CurrentSourceSwitches=off  DisableSnubberDevices=off  DisableRonSwitches=off  DisableVfSwitches=off  DisplayEquations=off  AutomaticDiscreteSolvers=off  SolverType=Tustin/Backward Euler (TBE)  Interpol=off  ExternalGateDelay=off  methode=off  Ts=100  x0status=blocks  SPID=on  SwTol=0  HookPort=off  NonlinearTolerance=1e-4  nMaxIteration=100  ContinueOnMaxIteration=off  RestoreLinks=warning  ResistiveCurrentMeasurement=off  Frange=[0:2:500]  Ylog=off  Xlog=on  ShowGrid=off  save=off  variable=ZData  structure=0  ZoomFFT=on  StartTime=0.0  cycles=1  DisplayStyle=1  fundamental=60  FreqAxis=off  MaxFrequency=1000  frequencyindicesteady=1  RmsSteady=1  display=off
  q : Constant  Value=1.6e-19
  I : Outport
  tag scope: I=global, V=global
  wires:
  [V] -> Add1/1
  [I] -> Divide4/1
  Divide4/1 -> Add1/2
  [Rs] -> Divide4/2
  Divide5/1 -> [Ish], Ish1/1
  Add1/1 -> Divide5/1
  [Rp] -> Divide5/2
  Add5/1 -> Divide15/2
  Divide15/1 -> [Iph], Id2/1
  Divide14/1 -> Add5/2
  [Top] -> Add10/1
  [KI] -> Divide14/1
  [Isc] -> Add5/1
  Add10/1 -> Divide14/2
  Divide13/1 -> [Id], Id1/1
  [n] -> Divide9/1
  [V] -> Divide29/1
  [I] -> Divide8/1
  Divide29/1 -> Add3/1
  [Rs] -> Divide8/2
  [Ns] -> Divide29/2
  Divide6/1 -> Math Function2/1
  Divide8/1 -> Add3/2
  [Ns] -> Divide8/3
  Constant3/1 -> Add4/2
  Math Function2/1 -> Add4/1
  Add3/1 -> Divide6/1
  [Np] -> Divide13/3
  [C] -> Divide9/3
  [Is] -> Divide13/2
  [Vt] -> Divide9/2
  Add4/1 -> Divide13/1
  Divide9/1 -> Divide6/2
  Math Function3/1 -> Divide3/2
  [n] -> Divide25/2
  Divide28/1 -> Math Function3/1
  Divide24/1 -> Divide28/2
  [k] -> Divide25/1
  Divide26/1 -> Add12/2
  Eg/1 -> Divide23/3
  [Tref] -> Divide27/2
  Divide3/1 -> Is/1, [Is]
  Constant5/1 -> Divide26/1
  Divide21/1 -> Divide22/2
  Divide25/1 -> Divide24/2
  Divide22/1 -> Divide3/1
  Divide20/1 -> Divide21/1, Divide21/2, Divide21/3
  [Irs] -> Divide22/1
  [Top] -> Divide26/2
  Divide23/1 -> Divide24/1
  [Tref] -> Divide20/2
  Divide27/1 -> Add12/1
  Add12/1 -> Divide28/1
  [q] -> Divide23/1, Divide23/2
  [Top] -> Divide20/1
  Constant6/1 -> Divide27/1
  Divide11/1 -> Mux/2, Power/1, To Workspace3/1, PV Graph/2
  [V] -> Mux/1
  Mux/1 -> To Workspace/1
  [I] -> Divide11/2, Mux/3, To Workspace2/1, Id4/1, IV Graph/2
  [V] -> Divide11/1, Id3/1, IV Graph/1, PV Graph/1, To Workspace1/1
  [Tref] -> Add10/2
  [Top] -> Divide18/3
  [n] -> Divide18/4
  Constant1/1 -> Add11/2
  Divide16/1 -> [Irs], Is2/1
  Math Function1/1 -> Add11/1
  Divide17/1 -> Divide19/1
  [q] -> Divide17/2
  Divide19/1 -> Math Function1/1
  [Isc] -> Divide16/1
  [C] -> Divide18/2
  Add11/1 -> Divide16/2
  [Voc] -> Divide17/1
  Divide18/1 -> Divide19/2
  [k] -> Divide18/1
  [Ish] -> Add6/2
  Add6/1 -> Scope3/1, Is1/1, I/1, [I]
  [Iph] -> Divide12/1
  [Np] -> Divide12/2
  Divide12/1 -> Add6/1
  [Id] -> Add6/3
  Isc/1 -> [Isc]
  [k] -> Divide/1
  k/1 -> [k]
  n/1 -> [n]
  Ns1/1 -> [Ns]
  [Top] -> Divide/2
  [q] -> Divide/3
  KV/1 -> [KV]
  KI/1 -> [KI]
  Temperature/1 -> [Tref]
  Np1/1 -> [Np]
  Rs/1 -> [Rs]
  Iro/1 -> [Iro]
  q/1 -> [q]
  G/1 -> [Irr], Scope/1
  Rp/1 -> [Rp]
  Divide/1 -> [Vt], Vt2/1
  cells in module/1 -> [C]
  Voc/1 -> [Voc]
  V/1 -> [V], Id5/1
  Top/1 -> [Top]
  [Irr] -> Divide1/1
  Divide1/1 -> Divide15/1
  Constant2/1 -> Divide1/2

== matlab function PV_ANN1/IoT_Node2 ==
  data: Vpv input; V_pv_iot2 output; Ipv input; G input; T input; t input; I_pv_iot2 output; G_solar_iot2 output; TxRate_iot2 output; Energy_iot2 output; Delay_iot2 output
function [V_pv_iot2, I_pv_iot2, G_solar_iot2,  ...
          TxRate_iot2, Energy_iot2, Delay_iot2] = IoT_Node2(Vpv, Ipv, G, T, t)
%============================================================
% IoT_Node2 – نود IoT شماره ۲ (نمونه‌برداری متوسط، نویز بالاتر)
%============================================================
Ts2     = 0.10;
noise2  = 0.015;
Ptx2    = 0.25;
P_idle  = 0.05; duty_tx = 0.10;
P_eq    = duty_tx*Ptx2 + (1-duty_tx)*P_idle;

persistent V_old I_old G_old T_old t_last E_old
if isempty(V_old)
    V_old = Vpv; I_old = Ipv; G_old = G; T_old = T; t_last = t; E_old = 0;
end

if t - t_last >= Ts2
    V_old = Vpv; I_old = Ipv; G_old = G; T_old = T;
    t_last = t; E_old = E_old + P_eq*Ts2;
end

Vn = V_old*(1+noise2*(2*rand-1));
In = I_old*(1+noise2*(2*rand-1));
Gn = G_old*(1+noise2*(2*rand-1));
Tn = T_old*(1+noise2*(2*rand-1));

V_pv_iot2 = quant(Vn,0,100,12);
I_pv_iot2 = quant(In,0,10,12);
G_solar_iot2 = quant(Gn,0,1200,12);
T_cell_iot2  = quant(Tn,0,80,12);

TxRate_iot2 = 1/Ts2;
Energy_iot2 = E_old;

Pkt_size = 512; Proc_t = 0.002; Net_jit = 0.001*rand;
Delay_tx = Pkt_size/(TxRate_iot2*1000);
Delay_iot2 = Delay_tx + Proc_t + Net_jit;
end

function yq = quant(y,ymin,ymax,Nbits)
levels = 2^Nbits-1;
y_clipped = min(max(y,ymin),ymax);
idx = round(((y_clipped-ymin)/(ymax-ymin))*levels);
yq = ymin + (idx/levels)*(ymax-ymin);
end

== matlab function PV_ANN1/IoT_Node3 ==
  data: Vpv input; V_pv_iot3 output; Ipv input; G input; T input; t input; I_pv_iot3 output; G_solar_iot3 output; TxRate_iot3 output; Energy_iot3 output; Delay_iot3 output
function [V_pv_iot3, I_pv_iot3, G_solar_iot3,  ...
          TxRate_iot3, Energy_iot3, Delay_iot3] = IoT_Node3(Vpv, Ipv, G, T, t)
%============================================================
% IoT_Node3 – نود IoT شماره ۳ (نمونه‌برداری آهسته، نویز زیاد)
%============================================================
Ts3     = 0.20;
noise3  = 0.02;
Ptx3    = 0.30;
P_idle  = 0.05; duty_tx = 0.10;
P_eq    = duty_tx*Ptx3 + (1-duty_tx)*P_idle;

persistent V_old I_old G_old T_old t_last E_old
if isempty(V_old)
    V_old = Vpv; I_old = Ipv; G_old = G; T_old = T; t_last = t; E_old = 0;
end

if t - t_last >= Ts3
    V_old = Vpv; I_old = Ipv; G_old = G; T_old = T;
    t_last = t; E_old = E_old + P_eq*Ts3;
end

Vn = V_old*(1+noise3*(2*rand-1));
In = I_old*(1+noise3*(2*rand-1));
Gn = G_old*(1+noise3*(2*rand-1));
Tn = T_old*(1+noise3*(2*rand-1));

V_pv_iot3 = quant(Vn,0,100,12);
I_pv_iot3 = quant(In,0,10,12);
G_solar_iot3 = quant(Gn,0,1200,12);
T_cell_iot3  = quant(Tn,0,80,12);

TxRate_iot3 = 1/Ts3;
Energy_iot3 = E_old;

Pkt_size = 512; Proc_t = 0.002; Net_jit = 0.001*rand;
Delay_tx = Pkt_size/(TxRate_iot3*1000);
Delay_iot3 = Delay_tx + Proc_t + Net_jit;
end

function yq = quant(y,ymin,ymax,Nbits)
levels = 2^Nbits-1;
y_clipped = min(max(y,ymin),ymax);
idx = round(((y_clipped-ymin)/(ymax-ymin))*levels);
yq = ymin + (idx/levels)*(ymax-ymin);
end

== matlab function PV_ANN1/5G_LinkModel1  ==
  data: Data_in input; SNR_dB output; IoT_rate input; Tx_Power_dBm input; d_m input; N0_dBmPerHz input; B_Hz input; MCS_index output; SE_eff output; Throughput_bps output; Delay_5G output; PacketLost output; Energy_5G output; MCS_in input
function [SNR_dB, MCS_index, SE_eff, Throughput_bps, ...
          Delay_5G, PacketLost, Energy_5G] = ...
    fcn(Data_in, IoT_rate, Tx_Power_dBm, d_m, N0_dBmPerHz, B_Hz, MCS_in)
%#codegen
% 5G uplink model for an IoT node:
% - Large-scale path loss (3GPP-like)
% - Small-scale Rayleigh (TDL-like)
% - Two modes for MCS:
%     (1) Internal SNR-based adaptation (baseline)
%     (2) External MCS input from ML/RL block
% - Simple PER, delay and energy model
%
% Inputs:
%   Data_in      : payload (packet length in bits, or vector)
%   IoT_rate     : packet generation rate from IoT layer [packet/s]
%   Tx_Power_dBm : transmit power [dBm]
%   d_m          : distance node–gNB [m]
%   N0_dBmPerHz  : noise PSD [dBm/Hz]
%   B_Hz         : bandwidth [Hz]
%   MCS_in       : (optional / از بیرون)
%                  - اگر خواستی MCS را ML تعیین کند → خروجی ML را اینجا بده
%                  - اگر نداشتی (یا -1 دادی) → داخل همین تابع بر اساس SNR انتخاب می‌شود

%% 0) Parameters (can be tuned)
G_BF_dB   = 10;      % Beamforming / antenna gain [dB]
modeURLLC = false;   % false: eMBB (~4 ms), true: URLLC (~1 ms)

%% 1) Distance & Path Loss (large-scale, with mobility)
d_km = d_m / 1000.0;
if d_km < 0.01
    d_km = 0.01;
end

% 3GPP TR 38.901 Urban Macro path loss (simplified, ~3.5 GHz)
PL_dB = 128.1 + 37.6*log10(d_km);

%% 2) Received power
Prx_dBm = Tx_Power_dBm + G_BF_dB - PL_dB;

%% 3) Noise power
N_dBm   = N0_dBmPerHz + 10*log10(B_Hz);      % dBm
SNR_dB_mean  = Prx_dBm - N_dBm;              % average SNR (no fading yet)
SNR_lin_mean = 10.^(SNR_dB_mean/10);

%% 4) Small-scale fading (TDL-like: few taps Rayleigh)

% Relative tap powers (dB) similar to a short TDL-C profile
p_dB  = [0 -2.2 -4 -6];
p_lin = 10.^(p_dB/10);

h2 = 0;
for k = 1:length(p_lin)
    re = randn;
    im = randn;
    alpha_k = sqrt(p_lin(k)/2) * (re + 1i*im);   % complex Gaussian tap
    h2 = h2 + abs(alpha_k)^2;
end

% Normalize so that E{|h|^2} ≈ 1
h2 = h2 / sum(p_lin);

SNR_lin = SNR_lin_mean * h2;
if SNR_lin < 1e-12
    SNR_lin = 1e-12;
end
SNR_dB = 10*log10(SNR_lin);

%% 5) MCS selection: internal (baseline) or external (ML/RL)

% جدول ثابت SE (همان جدول selectMCS_5G)
SNR_th = [-5  0   2   4   6   8   10  12  14  16  18  20  22  24];   % dB
SE_tab = [0.15 0.30 0.45 0.60 0.90 1.20 1.50 1.90 2.40 3.00 3.60 4.20 4.80 5.40];

use_external_MCS = (nargin >= 7) && ~isempty(MCS_in) && (~isnan(MCS_in));

if use_external_MCS
    % --- حالت ML/RL: از MCS_in استفاده کن ---
    mcs_idx = round(MCS_in);
    % clamp به بازه معتبر
    if mcs_idx < 0
        mcs_idx = 0;
    elseif mcs_idx > numel(SE_tab)-1
        mcs_idx = numel(SE_tab)-1;
    end
    SE_eff = SE_tab(mcs_idx+1);
else
    % --- حالت baseline: انتخاب MCS براساس SNR ---
    [mcs_idx, SE_eff] = selectMCS_5G_internal(SNR_dB, SNR_th, SE_tab);
end

MCS_index = mcs_idx;   % خروجی برای لاگ و رسم

%% 6) Throughput (bits per second)
% SE_eff: spectral efficiency [bit/s/Hz]
Throughput_bps = SE_eff * B_Hz;    % bit/s

% Packet length in bits
if numel(Data_in) == 1
    L_bits = Data_in;      % scalar = packet length
else
    L_bits = length(Data_in);
end

if Throughput_bps < 1
    Throughput_bps = 1;    % avoid division by zero
end

T_tx = L_bits / Throughput_bps;    % air time [s]

%% 7) Delay model (Tx time + queuing + processing)

% Processing delay (URLLC / eMBB)
if modeURLLC
    T_proc = 1e-3;         % 1 ms
else
    T_proc = 4e-3;         % 4 ms
end

% Inter-arrival time from IoT layer
if IoT_rate <= 0
    T_inter = 1e9;
else
    T_inter = 1 / IoT_rate;
end

T_queue = 0;
if T_tx > T_inter
    T_queue = T_tx - T_inter;
end

Delay_5G = T_tx + T_queue + T_proc;

%% 8) Packet Error Rate (PER) as function of SNR & MCS

PER = estimatePER_5G(SNR_dB, MCS_index);

u = rand;
if u < PER
    PacketLost = 1;
else
    PacketLost = 0;
end

%% 9) Energy consumption

Ptx_W   = 1e-3 * 10.^(Tx_Power_dBm/10);   % dBm -> W
Energy_5G = Ptx_W * T_tx;                 % Joule

end

% =====================================================================
%  Local functions
% =====================================================================

function [mcs_idx, SE_eff] = selectMCS_5G_internal(SNR_dB, SNR_th, SE_tab)
% Internal NR-like MCS table mapping SNR → (MCS, SE)

mcs_idx = 0;
SE_eff  = SE_tab(1);

for i = 1:length(SNR_th)
    if SNR_dB >= SNR_th(i)
        mcs_idx = i-1;       % MCS index (0-based)
        SE_eff  = SE_tab(i);
    else
        break;
    end
end

end

function PER = estimatePER_5G(SNR_dB, mcs_idx)
% Very simple PER model:
% better MCS (higher index) requires higher SNR.
% PER ≈ 1 / (1 + exp(a*(SNR - γ0))), with γ0 depending on MCS.

a = 0.9;                     % slope
gamma0 = -2 + 1.5*mcs_idx;   % required SNR increases with MCS index

PER = 1.0 ./ (1.0 + exp(a*(SNR_dB - gamma0)));

% clamp PER range
if PER < 1e-5
    PER = 1e-5;
elseif PER > 0.99
    PER = 0.99;
end

end

== matlab function PV_ANN1/5G_LinkModel 2 ==
  data: Data_in input; SNR_dB output; IoT_rate input; Tx_Power_dBm input; d_m input; N0_dBmPerHz input; B_Hz input; MCS_index output; SE_eff output; Throughput_bps output; Delay_5G output; PacketLost output; Energy_5G output; MCS_in input
function [SNR_dB, MCS_index, SE_eff, Throughput_bps, ...
          Delay_5G, PacketLost, Energy_5G] = ...
    fcn(Data_in, IoT_rate, Tx_Power_dBm, d_m, N0_dBmPerHz, B_Hz, MCS_in)
%#codegen
% 5G uplink model for an IoT node:
% - Large-scale path loss (3GPP-like)
% - Small-scale Rayleigh (TDL-like)
% - Two modes for MCS:
%     (1) Internal SNR-based adaptation (baseline)
%     (2) External MCS input from ML/RL block
% - Simple PER, delay and energy model
%
% Inputs:
%   Data_in      : payload (packet length in bits, or vector)
%   IoT_rate     : packet generation rate from IoT layer [packet/s]
%   Tx_Power_dBm : transmit power [dBm]
%   d_m          : distance node–gNB [m]
%   N0_dBmPerHz  : noise PSD [dBm/Hz]
%   B_Hz         : bandwidth [Hz]
%   MCS_in       : (optional / از بیرون)
%                  - اگر خواستی MCS را ML تعیین کند → خروجی ML را اینجا بده
%                  - اگر نداشتی (یا -1 دادی) → داخل همین تابع بر اساس SNR انتخاب می‌شود

%% 0) Parameters (can be tuned)
G_BF_dB   = 10;      % Beamforming / antenna gain [dB]
modeURLLC = false;   % false: eMBB (~4 ms), true: URLLC (~1 ms)

%% 1) Distance & Path Loss (large-scale, with mobility)
d_km = d_m / 1000.0;
if d_km < 0.01
    d_km = 0.01;
end

% 3GPP TR 38.901 Urban Macro path loss (simplified, ~3.5 GHz)
PL_dB = 128.1 + 37.6*log10(d_km);

%% 2) Received power
Prx_dBm = Tx_Power_dBm + G_BF_dB - PL_dB;

%% 3) Noise power
N_dBm   = N0_dBmPerHz + 10*log10(B_Hz);      % dBm
SNR_dB_mean  = Prx_dBm - N_dBm;              % average SNR (no fading yet)
SNR_lin_mean = 10.^(SNR_dB_mean/10);

%% 4) Small-scale fading (TDL-like: few taps Rayleigh)

% Relative tap powers (dB) similar to a short TDL-C profile
p_dB  = [0 -2.2 -4 -6];
p_lin = 10.^(p_dB/10);

h2 = 0;
for k = 1:length(p_lin)
    re = randn;
    im = randn;
    alpha_k = sqrt(p_lin(k)/2) * (re + 1i*im);   % complex Gaussian tap
    h2 = h2 + abs(alpha_k)^2;
end

% Normalize so that E{|h|^2} ≈ 1
h2 = h2 / sum(p_lin);

SNR_lin = SNR_lin_mean * h2;
if SNR_lin < 1e-12
    SNR_lin = 1e-12;
end
SNR_dB = 10*log10(SNR_lin);

%% 5) MCS selection: internal (baseline) or external (ML/RL)

% جدول ثابت SE (همان جدول selectMCS_5G)
SNR_th = [-5  0   2   4   6   8   10  12  14  16  18  20  22  24];   % dB
SE_tab = [0.15 0.30 0.45 0.60 0.90 1.20 1.50 1.90 2.40 3.00 3.60 4.20 4.80 5.40];

use_external_MCS = (nargin >= 7) && ~isempty(MCS_in) && (~isnan(MCS_in));

if use_external_MCS
    % --- حالت ML/RL: از MCS_in استفاده کن ---
    mcs_idx = round(MCS_in);
    % clamp به بازه معتبر
    if mcs_idx < 0
        mcs_idx = 0;
    elseif mcs_idx > numel(SE_tab)-1
        mcs_idx = numel(SE_tab)-1;
    end
    SE_eff = SE_tab(mcs_idx+1);
else
    % --- حالت baseline: انتخاب MCS براساس SNR ---
    [mcs_idx, SE_eff] = selectMCS_5G_internal(SNR_dB, SNR_th, SE_tab);
end

MCS_index = mcs_idx;   % خروجی برای لاگ و رسم

%% 6) Throughput (bits per second)
% SE_eff: spectral efficiency [bit/s/Hz]
Throughput_bps = SE_eff * B_Hz;    % bit/s

% Packet length in bits
if numel(Data_in) == 1
    L_bits = Data_in;      % scalar = packet length
else
    L_bits = length(Data_in);
end

if Throughput_bps < 1
    Throughput_bps = 1;    % avoid division by zero
end

T_tx = L_bits / Throughput_bps;    % air time [s]

%% 7) Delay model (Tx time + queuing + processing)

% Processing delay (URLLC / eMBB)
if modeURLLC
    T_proc = 1e-3;         % 1 ms
else
    T_proc = 4e-3;         % 4 ms
end

% Inter-arrival time from IoT layer
if IoT_rate <= 0
    T_inter = 1e9;
else
    T_inter = 1 / IoT_rate;
end

T_queue = 0;
if T_tx > T_inter
    T_queue = T_tx - T_inter;
end

Delay_5G = T_tx + T_queue + T_proc;

%% 8) Packet Error Rate (PER) as function of SNR & MCS

PER = estimatePER_5G(SNR_dB, MCS_index);

u = rand;
if u < PER
    PacketLost = 1;
else
    PacketLost = 0;
end

%% 9) Energy consumption

Ptx_W   = 1e-3 * 10.^(Tx_Power_dBm/10);   % dBm -> W
Energy_5G = Ptx_W * T_tx;                 % Joule

end

% =====================================================================
%  Local functions
% =====================================================================

function [mcs_idx, SE_eff] = selectMCS_5G_internal(SNR_dB, SNR_th, SE_tab)
% Internal NR-like MCS table mapping SNR → (MCS, SE)

mcs_idx = 0;
SE_eff  = SE_tab(1);

for i = 1:length(SNR_th)
    if SNR_dB >= SNR_th(i)
        mcs_idx = i-1;       % MCS index (0-based)
        SE_eff  = SE_tab(i);
    else
        break;
    end
end

end

function PER = estimatePER_5G(SNR_dB, mcs_idx)
% Very simple PER model:
% better MCS (higher index) requires higher SNR.
% PER ≈ 1 / (1 + exp(a*(SNR - γ0))), with γ0 depending on MCS.

a = 0.9;                     % slope
gamma0 = -2 + 1.5*mcs_idx;   % required SNR increases with MCS index

PER = 1.0 ./ (1.0 + exp(a*(SNR_dB - gamma0)));

% clamp PER range
if PER < 1e-5
    PER = 1e-5;
elseif PER > 0.99
    PER = 0.99;
end

end
